simulink model "realmsanores"  (R2013a)
settings: Solver=ode45  StartTime=0.0  StopTime=600  RelTol=1e-3
undefined symbols (not defined in the file or in its folder): Ensamblaje3, masa2, Pieza2, Pieza4, RootGround, RootPart
libraries: mblibv1 x14
settings Model: Creator=oiluj  LastModifiedBy=Daniel
settings OptimizationCC: ExpressionDepthLimit=2147483647
settings SimMechanicsCC: VisOnUpdateDiagram=on  VisDuringSimulation=on

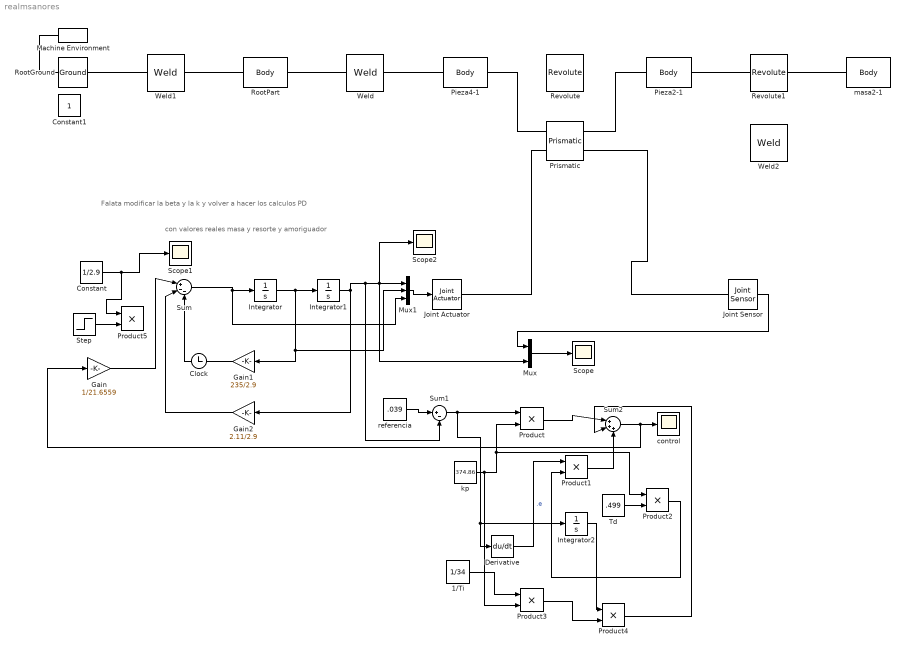
== system realmsanores ==
  note: con valores reales masa y resorte y amoriguador
  note: Falata modificar la beta y la k y volver a hacer los calculos PD
  1/Ti : Constant  Value=1/34
  Constant : Constant  Value=1/2.9
  Derivative : Derivative
  Gain : Gain  Gain=1/21.6559
  Gain1 : Gain  Gain=235/2.9
  Gain2 : Gain  Gain=2.11/2.9
  Integrator : Integrator
  Integrator1 : Integrator
  Integrator2 : Integrator
  Joint Actuator : mblibv1/Sensors &  Actuators/Joint Actuator  UpdateFromCAD=off  PhysicalDomain=Mechanical  PortType=blob  ActuationStyle=Motion  AngleUnits=deg  ArcVelocityUnits=deg/s  ArcAccelerationUnits=deg/s^2  CoordPositionUnits=m  VelocityUnits=m/s  AccelerationUnits=m/s^2  ForceUnits=mN  TorqueUnits=N*m  ActiveIO=on  Width=3  DialogClass=MechanicalActuatorBlock  Primitive=P1  ReferenceFrame=Absolute (World)
  Joint Sensor : mblibv1/Sensors &  Actuators/Joint Sensor  UpdateFromCAD=off  PhysicalDomain=Mechanical  PortType=blob  Muxed=off  Pose=off  Angle=on  AngleUnits=deg  ArcVelocity=off  ArcVelocityUnits=deg/s  ArcAcceleration=off  ArcAccelerationUnits=deg/s^2  CoordPosition=on  CoordPositionUnits=m  Velocity=off  VelocityUnits=m/s  Acceleration=off  AccelerationUnits=m/s^2  Quaternion=on  QuaternionDT=off  QuaternionDDT=off  QuaternionUnits=off  OutputVector=[1]  ActiveIO=on  Width=1  DialogClass=MechanicalSensorBlock  Primitive=P1  Force=off  ForceUnits=N  Torque=off  TorqueUnits=N*m  ReferenceFrame=Absolute (World)  ReactionSensedSide=Base  ReactionReferenceFrame=Absolute (World)  ReactionForce=off  ReactionForceUnits=N  ReactionMoment=off  ReactionMomentUnits=N*m
  Machine Environment : mblibv1/Bodies/Machine Environment  PortType=env  PhysicalDomain=Mechanical  DialogTemplateClass=MECH.MachineEnvironment  SyncWhenCopied=off  Gravity=[0 -9.81 0]  GravityUnits=m/s^2  GravityAsSignal=off  Dimensionality=Auto-detect  AnalysisType=Forward dynamics  LinearAssemblyTolerance=1e-3  LinearAssemblyToleranceUnits=m  AngularAssemblyTolerance=1e-3  AngularAssemblyToleranceUnits=rad  ConstraintSolverType=Stabilizing  ConstraintRelTolerance=1e-4  ConstraintAbsTolerance=1e-4  UseRobustSingularityHandling=off  RedundancyAnalysisToleranceType=Automatically select tolerance  RedundancyAnalysisTolerance=1e-14  StatePerturbationType=Fixed  PerturbationSize=1e-5  VisualizeMachine=on  BodyVisualizationType=Use model default body geometries  BodyColorSelMode=Use model default  DefaultBodyColor=[1 0 0]
  Mux : Mux  Inputs=2
  Mux1 : Mux  Inputs=3
  Pieza2-1 : mblibv1/Bodies/Body  LConnTagsString=CS2  RConnTagsString=CS3  UpdateFromCAD=on  PMImportedID=Pieza2-1  DialogClass=MechanicalBodyBlock  Mass=1.96575  MassUnits=kg  InertiaUnits=kg*m^2  Inertia=[0.00655307,-0.000148207,9.87728e-07;-0.000148207,0.00488642,4.3422e-07;9.87728e-07,4.3422e-07,0.00661981]  Shape=Cylinder  ShapeDims=[1 1]  ShapeUnits=m  ShapeUse=false  Density=1  DensityUnits=kg/m^3  DensityUse=false  GraphicsMode=GFXFILE  GraphicsFileName=Ensamblaje3 - Pieza2-1.STL  BodyColorSelMode=COLORPALETTE  BodyColor=[0.647059;0.619608;0.588235]  AttachedToCS=CS1  CG=Right$CG$[-3.075e-05 0.0905504 0.106824]$WORLD$WORLD$m$[-0.36166 0 -0.93231;0 1 0;0.93231 0 -0.36166]$3x3 Transform$rad$WORLD$false$Pieza2-1::CG(AUTOGEN)  WorkingFrames=Right$CS1$[0.00166441 0.0153865 0.107587]$WORLD$WORLD$m$[-0.36166 0 -0.93231;0 1 0;0.93231 0 -0.36166]$3x3 Transform$rad$WORLD$false$Pieza2-1::CS1(AUTOGEN)#Left$CS2$[-0.00120571 -0.0101135 0.1]$WORLD$WORLD$m$[1 0 0;0 1 0;0 0 1]$3x3 Transform$rad$WORLD$true$Pieza2-1:-:Pieza4-1::Pieza2-1(AUTOGEN)#Right$CS3$[-0.00156332 0.189587 0.102083]$WORLD$WORLD$m$[1 0 0;0 1 0;0 0 1]$3x3 Transform$rad$WORLD$true$Pieza2-1:-:masa2-1::Pieza2-1(AUTOGEN)  CGPos=[-3.075e-05 0.0905504 0.106824]  CGRot=[-0.36166 0 -0.93231;0 1 0;0.93231 0 -0.36166]  CS0Pos=[]  CS0Rot=[]  CS1Pos=[0.00166441 0.0153865 0.107587]  CS1Rot=[-0.36166 0 -0.93231;0 1 0;0.93231 0 -0.36166]  CS2Pos=[-0.00120571 -0.0101135 0.1]  CS2Rot=[1 0 0;0 1 0;0 0 1]  CS3Pos=[-0.00156332 0.189587 0.102083]  CS3Rot=[1 0 0;0 1 0;0 0 1]  CS4Pos=[]  CS4Rot=[]  CS5Pos=[]  CS5Rot=[]  CS6Pos=[]  CS6Rot=[]  CS7Pos=[]  CS7Rot=[]  CS8Pos=[]  CS8Rot=[]  CS9Pos=[]  CS9Rot=[]  CS10Pos=[]  CS10Rot=[]  CS11Pos=[]  CS11Rot=[]  CS12Pos=[]  CS12Rot=[]  CS13Pos=[]  CS13Rot=[]  CS14Pos=[]  CS14Rot=[]  CS15Pos=[]  CS15Rot=[]  CS16Pos=[]  CS16Rot=[]  CS17Pos=[]  CS17Rot=[]  CS18Pos=[]  CS18Rot=[]  CS19Pos=[]  CS19Rot=[]  CS20Pos=[]  CS20Rot=[]
  Pieza4-1 : mblibv1/Bodies/Body  LConnTagsString=CS2  RConnTagsString=CS3  UpdateFromCAD=on  PMImportedID=Pieza4-1  DialogClass=MechanicalBodyBlock  Mass=1.0279  MassUnits=kg  InertiaUnits=kg*m^2  Inertia=[0.000852582,0,0;0,0.00166789,0;0,0,0.000852582]  Shape=Cylinder  ShapeDims=[1 1]  ShapeUnits=m  ShapeUse=false  Density=1  DensityUnits=kg/m^3  DensityUse=false  GraphicsMode=GFXFILE  GraphicsFileName=Ensamblaje3 - Pieza4-1.STL  BodyColorSelMode=COLORPALETTE  BodyColor=[0.2;0.2;0.2]  AttachedToCS=CS1  CG=Right$CG$[-0.00120571 -0.0128214 0.1]$WORLD$WORLD$m$[1 0 0;0 1 0;0 0 1]$3x3 Transform$rad$WORLD$false$Pieza4-1::CG(AUTOGEN)  WorkingFrames=Right$CS1$[-0.0512057 -0.0201135 0.15]$WORLD$WORLD$m$[1 0 0;0 1 0;0 0 1]$3x3 Transform$rad$WORLD$false$Pieza4-1::CS1(AUTOGEN)#Left$CS2$[-0.00120571 -0.0128214 0.1]$WORLD$WORLD$m$[1 0 0;0 1 0;0 0 1]$3x3 Transform$rad$WORLD$true$Ensamblaje3/RootPart:-:Pieza4-1::Pieza4-1(AUTOGEN)#Right$CS3$[-0.00120571 -0.0101135 0.1]$WORLD$WORLD$m$[1 0 0;0 1 0;0 0 1]$3x3 Transform$rad$WORLD$true$Pieza2-1:-:Pieza4-1::Pieza4-1(AUTOGEN)  CGPos=[-0.00120571 -0.0128214 0.1]  CGRot=[1 0 0;0 1 0;0 0 1]  CS0Pos=[]  CS0Rot=[]  CS1Pos=[-0.0512057 -0.0201135 0.15]  CS1Rot=[1 0 0;0 1 0;0 0 1]  CS2Pos=[-0.00120571 -0.0128214 0.1]  CS2Rot=[1 0 0;0 1 0;0 0 1]  CS3Pos=[-0.00120571 -0.0101135 0.1]  CS3Rot=[1 0 0;0 1 0;0 0 1]  CS4Pos=[]  CS4Rot=[]  CS5Pos=[]  CS5Rot=[]  CS6Pos=[]  CS6Rot=[]  CS7Pos=[]  CS7Rot=[]  CS8Pos=[]  CS8Rot=[]  CS9Pos=[]  CS9Rot=[]  CS10Pos=[]  CS10Rot=[]  CS11Pos=[]  CS11Rot=[]  CS12Pos=[]  CS12Rot=[]  CS13Pos=[]  CS13Rot=[]  CS14Pos=[]  CS14Rot=[]  CS15Pos=[]  CS15Rot=[]  CS16Pos=[]  CS16Rot=[]  CS17Pos=[]  CS17Rot=[]  CS18Pos=[]  CS18Rot=[]  CS19Pos=[]  CS19Rot=[]  CS20Pos=[]  CS20Rot=[]
  Prismatic : mblibv1/Joints/Prismatic  LConnTagsString=__newl0|SA1  RConnTagsString=__newr0|SA1  UpdateFromCAD=off  NumSAPorts=2  CutJoint=off  MarkAsCut=off  Primitives=prismatic  PrimitiveProps=P1$World$[0 1 0]$prismatic  DialogClass=JointBlock  P1Axis=[0 1 0]
  Product{,1..5} (6 alike) : Product
  Revolute : mblibv1/Joints/Revolute  LConnTagsString=__newl0  RConnTagsString=__newr0  UpdateFromCAD=on  PMImportedID=Pieza2-1:-:Pieza4-1  NumSAPorts=0  CutJoint=off  MarkAsCut=off  Primitives=prismatic  PrimitiveProps=R1$WORLD$[0,1,0]$revolute  DialogClass=JointBlock  R1Axis=[0,1,0]
  Revolute1 : mblibv1/Joints/Revolute  LConnTagsString=__newl0  RConnTagsString=__newr0  UpdateFromCAD=on  PMImportedID=Pieza2-1:-:masa2-1  NumSAPorts=0  CutJoint=off  MarkAsCut=off  Primitives=prismatic  PrimitiveProps=R1$WORLD$[0,-1,0]$revolute  DialogClass=JointBlock  R1Axis=[0,-1,0]
  RootGround : mblibv1/Bodies/Ground  UpdateFromCAD=on  PMImportedID=RootGround  LeftPortType=env  RightPortType=workingframe  PhysicalDomain=Mechanical  DialogClass=GroundBlock  CoordPosition=[-0.00142619,0.265503,0.102374]  CoordPositionUnits=m  StateVectorMgrId=-1  MachineId=[0 0]  ShowEnvPort=on
  RootPart : mblibv1/Bodies/Body  LConnTagsString=CS3  RConnTagsString=CS2  UpdateFromCAD=on  PMImportedID=Ensamblaje3/RootPart  DialogClass=MechanicalBodyBlock  Mass=0  MassUnits=kg  InertiaUnits=kg*m^2  Inertia=[0,0,0;0,0,0;0,0,0]  Shape=Cylinder  ShapeDims=[1 1]  ShapeUnits=m  ShapeUse=false  Density=1  DensityUnits=kg/m^3  DensityUse=false  GraphicsMode=MACHINE_DEFAULT  BodyColorSelMode=MACHINE_DEFAULT  BodyColor=[1;0;0]  AttachedToCS=CS1  CG=Right$CG$[-0.00142619 0.265503 0.102374]$WORLD$WORLD$m$[1 0 0;0 1 0;0 0 1]$3x3 Transform$rad$WORLD$false$Ensamblaje3/RootPart::CG(AUTOGEN)  WorkingFrames=Right$CS1$[0 0 0]$WORLD$WORLD$m$[1 0 0;0 1 0;0 0 1]$3x3 Transform$rad$WORLD$false$Ensamblaje3/RootPart::CS1(AUTOGEN)#Right$CS2$[-0.00120571 -0.0128214 0.1]$WORLD$WORLD$m$[1 0 0;0 1 0;0 0 1]$3x3 Transform$rad$WORLD$true$Ensamblaje3/RootPart:-:Pieza4-1::Ensamblaje3/RootPart(AUTOGEN)#Left$CS3$[-0.00142619 0.265503 0.102374]$WORLD$WORLD$m$[1 0 0;0 1 0;0 0 1]$3x3 Transform$rad$WORLD$true$Ensamblaje3/RootPart:-:RootGround::Ensamblaje3/RootPart(AUTOGEN)  CGPos=[-0.00142619 0.265503 0.102374]  CGRot=[1 0 0;0 1 0;0 0 1]  CS0Pos=[]  CS0Rot=[]  CS1Pos=[0 0 0]  CS1Rot=[1 0 0;0 1 0;0 0 1]  CS2Pos=[-0.00120571 -0.0128214 0.1]  CS2Rot=[1 0 0;0 1 0;0 0 1]  CS3Pos=[-0.00142619 0.265503 0.102374]  CS3Rot=[1 0 0;0 1 0;0 0 1]  CS4Pos=[]  CS4Rot=[]  CS5Pos=[]  CS5Rot=[]  CS6Pos=[]  CS6Rot=[]  CS7Pos=[]  CS7Rot=[]  CS8Pos=[]  CS8Rot=[]  CS9Pos=[]  CS9Rot=[]  CS10Pos=[]  CS10Rot=[]  CS11Pos=[]  CS11Rot=[]  CS12Pos=[]  CS12Rot=[]  CS13Pos=[]  CS13Rot=[]  CS14Pos=[]  CS14Rot=[]  CS15Pos=[]  CS15Rot=[]  CS16Pos=[]  CS16Rot=[]  CS17Pos=[]  CS17Rot=[]  CS18Pos=[]  CS18Rot=[]  CS19Pos=[]  CS19Rot=[]  CS20Pos=[]  CS20Rot=[]
  Scope : Scope
  Scope1 : Scope
      settings: YMin=0.033158  YMax=0.0366484  SaveName=ScopeData3
  Scope2 : Scope
      settings: YMin=0.033158  YMax=0.0366484  SaveName=chi
  Step : Step  SampleTime=0
  Sum : Sum  Inputs=|+--
  Sum1 : Sum  Inputs=|+-
  Sum2 : Sum  Inputs=|+++
  Td : Constant  Value=.499
  Weld : mblibv1/Joints/Weld  LConnTagsString=__newl0  RConnTagsString=__newr0  UpdateFromCAD=on  PMImportedID=Ensamblaje3/RootPart:-:Pieza4-1  NumSAPorts=0  CutJoint=off  MarkAsCut=off  Primitives=weld  PrimitiveProps=W$WORLD$[0.57735,0.57735,0.57735]$weld  DialogClass=JointBlock  WAxis=[0.57735,0.57735,0.57735]
  Weld1 : mblibv1/Joints/Weld  LConnTagsString=__newl0  RConnTagsString=__newr0  UpdateFromCAD=on  PMImportedID=Ensamblaje3/RootPart:-:RootGround  NumSAPorts=0  CutJoint=off  MarkAsCut=off  Primitives=weld  PrimitiveProps=W$WORLD$[0.57735,0.57735,0.57735]$weld  DialogClass=JointBlock  WAxis=[0.57735,0.57735,0.57735]
  Weld2 : mblibv1/Joints/Weld  LConnTagsString=__newl0  RConnTagsString=__newr0  UpdateFromCAD=on  NumSAPorts=0  CutJoint=off  MarkAsCut=off  Primitives=weld  PrimitiveProps=W$WORLD$[0.57735,0.57735,0.57735]$weld  DialogClass=JointBlock  WAxis=[0.57735,0.57735,0.57735]
  control : Scope
      settings: YMin=77.5  YMax=84
  kp : Constant  Value=374.86
  masa2-1 : mblibv1/Bodies/Body  LConnTagsString=CS2  UpdateFromCAD=on  PMImportedID=masa2-1  DialogClass=MechanicalBodyBlock  Mass=21.6559  MassUnits=kg  InertiaUnits=kg*m^2  Inertia=[0.190928,0,0;0,0.190945,0;0,0,0.190928]  Shape=Cylinder  ShapeDims=[1 1]  ShapeUnits=m  ShapeUse=false  Density=1  DensityUnits=kg/m^3  DensityUse=false  GraphicsMode=GFXFILE  GraphicsFileName=Ensamblaje3 - masa2-1.STL  BodyColorSelMode=COLORPALETTE  BodyColor=[1 1 1]  AttachedToCS=CS1  CG=Right$CG$[-0.00156332 0.294595 0.102083]$WORLD$WORLD$m$[-0.94926 0 0.314493;0 -1 0;0.314493 0 0.94926]$3x3 Transform$rad$WORLD$false$masa2-1::CG(AUTOGEN)  WorkingFrames=Right$CS1$[0.143768 0.409587 0.175081]$WORLD$WORLD$m$[-0.94926 0 0.314493;0 -1 0;0.314493 0 0.94926]$3x3 Transform$rad$WORLD$false$masa2-1::CS1(AUTOGEN)#Left$CS2$[-0.00156332 0.189587 0.102083]$WORLD$WORLD$m$[1 0 0;0 1 0;0 0 1]$3x3 Transform$rad$WORLD$true$Pieza2-1:-:masa2-1::masa2-1(AUTOGEN)  CGPos=[-0.00156332 0.294595 0.102083]  CGRot=[-0.94926 0 0.314493;0 -1 0;0.314493 0 0.94926]  CS0Pos=[]  CS0Rot=[]  CS1Pos=[0.143768 0.409587 0.175081]  CS1Rot=[-0.94926 0 0.314493;0 -1 0;0.314493 0 0.94926]  CS2Pos=[-0.00156332 0.189587 0.102083]  CS2Rot=[1 0 0;0 1 0;0 0 1]  CS3Pos=[]  CS3Rot=[]  CS4Pos=[]  CS4Rot=[]  CS5Pos=[]  CS5Rot=[]  CS6Pos=[]  CS6Rot=[]  CS7Pos=[]  CS7Rot=[]  CS8Pos=[]  CS8Rot=[]  CS9Pos=[]  CS9Rot=[]  CS10Pos=[]  CS10Rot=[]  CS11Pos=[]  CS11Rot=[]  CS12Pos=[]  CS12Rot=[]  CS13Pos=[]  CS13Rot=[]  CS14Pos=[]  CS14Rot=[]  CS15Pos=[]  CS15Rot=[]  CS16Pos=[]  CS16Rot=[]  CS17Pos=[]  CS17Rot=[]  CS18Pos=[]  CS18Rot=[]  CS19Pos=[]  CS19Rot=[]  CS20Pos=[]  CS20Rot=[]
  referencia : Constant  Value=.039
  Clock : Clock
      settings: IOType=siggen
  Constant1 : Constant  IOType=siggen
  wires:
  Sum2/1 -> Gain/1, control/1
  Gain1/1 -> Sum/3
  Gain2/1 -> Sum/2
  Sum/1 -> Integrator/1, Mux1/3
  Integrator/1 -> Integrator1/1, Gain1/1, Mux1/2
  Mux/1 -> Scope/1
  Joint Sensor/1 -> Mux/1
  Mux1/1 -> Joint Actuator/1
  referencia/1 -> Sum1/1
  Sum1/1 -> Integrator2/1, Derivative/1, Product/1
  kp/1 -> Product/2, Product2/1, Product3/2
  Product/1 -> Sum2/1
  Product2/1 -> Product1/2
  Td/1 -> Product2/2
  Derivative/1 -> Product1/1  ".e"
  Integrator1/1 -> Gain2/1, Sum1/2, Mux/2, Scope2/1, Mux1/1
  1/Ti/1 -> Product3/1
  Product3/1 -> Product4/2
  Integrator2/1 -> Product4/1
  Product1/1 -> Sum2/3
  Constant/1 -> Product5/1, Scope1/1
  Step/1 -> Product5/2
  Product4/1 -> Sum2/2
  Gain/1 -> Sum/1
  connections:
  RootPart/RConn1 -- Weld/LConn1
  Weld/RConn1 -- Pieza4-1/LConn1
  Pieza4-1/RConn1 -- Prismatic/LConn1
  Prismatic/RConn1 -- Pieza2-1/LConn1
  Pieza2-1/RConn1 -- Revolute1/LConn1
  Revolute1/RConn1 -- masa2-1/LConn1
  RootGround/RConn1 -- Weld1/LConn1
  Weld1/RConn1 -- RootPart/LConn1
  RootGround/LConn1 -- Machine Environment/RConn1
  Joint Actuator/RConn1 -- Prismatic/LConn2
  Joint Sensor/LConn1 -- Prismatic/RConn2
